simulink model "samplingSystem"  (R2018b)
settings: Solver=VariableStepAuto  StartTime=0.0  StopTime=200  RelTol=1e-3
settings Model: Creator=nmass  LastModifiedBy=nmass

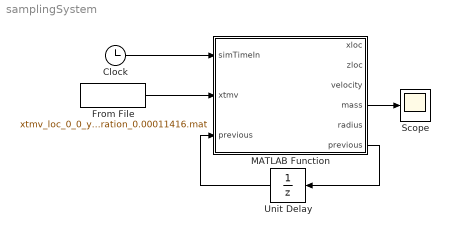
== system samplingSystem ==
  Clock : Clock
  From File : FromFile  FileName=xtmv_loc_0_0_year_2020_duration_0.00011416.mat  SampleTime=0  ExtrapolationBeforeFirstDataPoint=Ground value  InterpolationWithinTimeRange=Zero order hold  ExtrapolationAfterLastDataPoint=Hold last value
  MATLAB Function : MATLAB Function  TreatAsAtomicUnit=on
  Scope : Scope
  Unit Delay : UnitDelay  SampleTime=-1
  wires:
  Clock/1 -> MATLAB Function/1(simTimeIn)
  From File/1 -> MATLAB Function/2(xtmv)
  MATLAB Function/6(previous) -> Unit Delay/1
  Unit Delay/1 -> MATLAB Function/3("previous ")
  MATLAB Function/4(mass) -> Scope/1

== matlab function samplingSystem/MATLAB Function ==
  data: xloc output; zloc output; simTimeIn input; velocity output; xtmv input; mass output; radius output; previous input; previous output
function [xloc, zloc, velocity, mass, radius, previous] = meteoroidSampler(simTimeIn, xtmv, previous)
    % This matlab block takes in the sim time and returns an impact
    % only once when relevant. values are UNDEFINED otherwise.
    UNDEFINED = 0;
    % this is the mean density, ill adjust the program to output real
    % densities later
    density = 1.83; %g/cm^2
    
    % Set inital values
    velocity = [UNDEFINED,UNDEFINED,UNDEFINED];
    mass = UNDEFINED;
    radius = UNDEFINED;
    xloc = UNDEFINED;
    zloc = UNDEFINED;
    
    if (xtmv(3) <= simTimeIn) && (abs(previous - xtmv(4)/1000) > 0.0000000001)
        % If the sim time has passed an impact, and the impact has not been
        % reported yet, send it out.
        
        % use the defined habitat coordinate system
        xloc = xtmv(2);
        zloc = xtmv(1);
        x = xtmv(5);
        y = xtmv(6);
        z = xtmv(7);
        velocity = [y,z,x];
        
        % Mass values
        mass = xtmv(4) / 1000; % convert from g to kg
        previous = mass;
        % backwards calculate radius from density and mass
        radius = (3 * mass * 1000 / ( 4 * pi * density))^(1/3);
        radius = radius / 100; % cm to m
        
    else
        % return all zeros and prev as the previous mass
        return;
    end 
    %fprintf("%f %f %f\n", simTimeIn, prev, mass);
end
